simulink model "adm1"  (Simulink 6.1)
settings: Solver=ode15s  SolverMode=SingleTasking  StartTime=0.0  StopTime=600  MaxStep=0.5  RelTol=1e-6  AbsTol=1e-6
PreLoadFcn:
  | ADM1init
libraries: simulink x1
settings Model: Creator=ielulf  LastModifiedBy=evren.tugtas  ExtModeTrigMode=oneshot  ExtModeArmWhenConnect=off  ExtModeAutoUpdateStatusClock=off
settings DataIOCC: LimitDataPoints=off  SignalLoggingName=sigsOut
settings OptimizationCC: BlockReduction=off  BooleanDataType=off
settings HardwareCC: TargetUnknown=on
settings GRTTargetCC: ModelReferenceCompliant=off  MatFileLogging=off

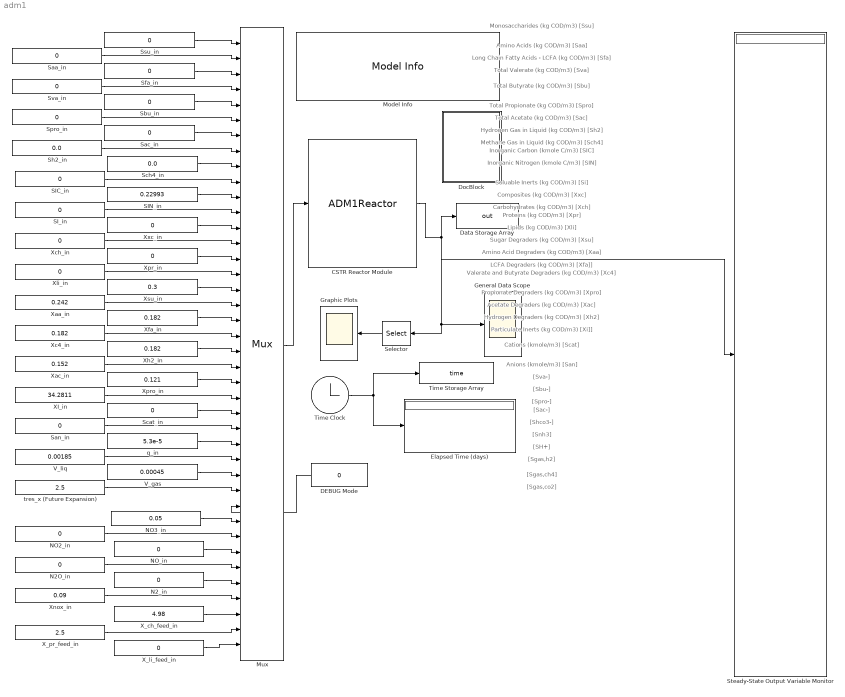
== system adm1 ==
  note: Monosaccharides (kg COD/m3) [Ssu]
  note: Amino Acids (kg COD/m3) [Saa]
  note: Long Chain Fatty Acids - LCFA (kg COD/m3) [Sfa]
  note: Total Valerate (kg COD/m3) [Sva]
  note: Total Butyrate (kg COD/m3) [Sbu]
  note: Total Propionate (kg COD/m3) [Spro]
  note: Total Acetate (kg COD/m3) [Sac]
  note: Hydrogen Gas in Liquid (kg COD/m3) [Sh2]
  note: Methane Gas in Liquid (kg COD/m3) [Sch4]
  note: Inorganic Carbon (kmole C/m3) [SIC]
  note: Inorganic Nitrogen (kmole C/m3) [SIN]
  note: Soluable Inerts (kg COD/m3) [Si]
  note: Composites (kg COD/m3) [Xxc]
  note: Carbohydrates (kg COD/m3) [Xch]
  note: Proteins (kg COD/m3) [Xpr]
  note: Lipids (kg COD/m3) [Xli]
  note: Amino Acid Degraders (kg COD/m3) [Xaa]
  note: LCFA Degraders (kg COD/m3) [Xfa]]
  note: Valerate and Butyrate Degraders (kg COD/m3) [Xc4]
  note: Propionate Degraders (kg COD/m3) [Xpro]
  note: Acetate Degraders (kg COD/m3) [Xac]
  note: Hydrogen Degraders (kg COD/m3) [Xh2]
  note: Particulate Inerts (kg COD/m3) [Xi]]
  note: Cations (kmole/m3) [Scat]
  note: Anions (kmole/m3) [San]
  note: [Sva-]
  note: [Sbu-]
  note: [Spro-]
  note: [Sac-]
  note: [Shco3-]
  note: [Snh3]
  note: [SH+]
  note: [Sgas,h2]
  note: [Sgas,ch4]
  note: [Sgas,co2]
  note: Sugar Degraders (kg COD/m3) [Xsu]
  CSTR Reactor Module : S-Function  FunctionName=ADM1Reactor
  DEBUG Mode : Constant  Tag=DEBUG  Orientation=left  Priority=0  Value=0  OutDataTypeMode=double
  Data Storage Array : ToWorkspace  VariableName=out  SampleTime=-1  SaveFormat=Array
      settings: Priority=14
  DocBlock : Subsystem  mask(DocBlock){ECoderFlag=, DocumentType=Text}
      mask prompts: ECoderFlag "E Coder Flag"; DocumentType "Document Type"
      mask help: Use this block to save long descriptive text with the model. Double-clicking the block will open an editor.
      settings: CopyFcn=docblock('breaklink',gcb);  DeleteFcn=docblock('close_document',gcb);  PreSaveFcn=docblock('save_document',gcb);  OpenFcn=docblock('edit_document',gcb);
      mask StyleString: edit,popup(Text|RTF|HTML)
      mask Display:
      | plot([.8 0 0 1 1 .8 .8 1],[1 1 0 0 .8 1 .8 .8]);
      | text(.5,.5,'DOC','horizontalalignment','center');
  Elapsed Time (days) : Display
      settings: Priority=4
  General Data Scope : Scope
      settings: TickLabels=on  YMin=0  YMax=50  SaveName=N1  DataFormat=Structure
  Graphic Plots : Scope
      settings: TickLabels=on  YMin=0.1  YMax=0.32  SaveName=N  DataFormat=Array
  Model Info : simulink/Model-Wide Utilities/Model Info  InitialBlockCM=none  BlockCM=none  Frame=on  DisplayStringWithTags=|  HorizontalTextAlignment=Left  LeftAlignmentValue=0.02  SourceBlockDiagram=adm1  TagMaxNumber=20
      | ADM1 Anaerobic Digestion Model %<Description>
      | Date Created: %<Created>
      | Date Last Modification: %<ModifiedDate>
      | Last Modified By: %<ModifiedBy>
      | ADM1 Model Version: %<ModelVersion>
      | ON-LINE DOCUMENTATION MANUAL  ===V=V=V=== %<ModifiedComment>
  Mux : Mux  Inputs=40
  N2O_in : Constant  Tag=N2O_in  Priority=0  Value=0  OutDataTypeMode=double
  N2_in : Constant  Tag=N2_in  Priority=0  Value=0  OutDataTypeMode=double
  NO2_in : Constant  Tag=NO2_in  Priority=0  Value=0  OutDataTypeMode=double
  NO3_in : Constant  Tag=NO3_in  Priority=0  Value=0.05  OutDataTypeMode=double
  NO_in : Constant  Tag=NO_in  Priority=0  Value=0  OutDataTypeMode=double
  SIC_in : Constant  Tag=SIC_in  Priority=0  Value=0  OutDataTypeMode=double
  SIN_in : Constant  Tag=SIN_in  Priority=0  Value=0.22993  OutDataTypeMode=double
  SI_in : Constant  Tag=SI_in  Priority=0  Value=0  OutDataTypeMode=double
  Saa_in : Constant  Tag=Saa_in  Priority=0  Value=0  OutDataTypeMode=double
  Sac_in : Constant  Tag=Sac_in  Priority=0  Value=0  OutDataTypeMode=double
  San_in : Constant  Tag=San_in  Priority=0  Value=0  OutDataTypeMode=double
  Sbu_in : Constant  Tag=Sbu_in  Priority=0  Value=0  OutDataTypeMode=double
  Scat_in : Constant  Priority=0  Value=0  OutDataTypeMode=double
  Sch4_in : Constant  Tag=Sch4_in  Priority=0  Value=0.0  OutDataTypeMode=double
  Selector : Selector  Orientation=left  Elements="[1  2  3  4  5  6  7]"  InputPortWidth=48
      settings: OpenFcn=ADM1Output
  Sfa_in : Constant  Tag=Sfa_in  Priority=0  Value=0  OutDataTypeMode=double
  Sh2_in : Constant  Tag=Sh2_in  Priority=0  Value=0.0  OutDataTypeMode=double
  Spro_in : Constant  Tag=Spro_in  Priority=0  Value=0  OutDataTypeMode=double
  Ssu_in : Constant  Tag=Ssu_in  Priority=0  Value=0  OutDataTypeMode=double
  Steady-State Output Variable Monitor : Display
      settings: Priority=2
  Sva_in : Constant  Tag=Sva_in  Priority=0  Value=0  OutDataTypeMode=double
  Time Clock : Clock
      settings: Priority=3  Decimation=10
  Time Storage Array : ToWorkspace  VariableName=time  SampleTime=-1  SaveFormat=Array
      settings: Priority=5
  V_gas : Constant  Tag=V_gas  Priority=0  Value=0.00045  OutDataTypeMode=double
  V_liq : Constant  Tag=V_liq  Priority=0  Value=0.00185  OutDataTypeMode=double
  XI_in : Constant  Tag=XI_in  Priority=0  Value=34.2811  OutDataTypeMode=double
  X_ch_feed_in : Constant  Tag=X_ch_feed_in  Priority=0  Value=4.98  OutDataTypeMode=double
  X_li_feed_in : Constant  Tag=X_li_feed_in  Priority=0  Value=0  OutDataTypeMode=double
  X_pr_feed_in : Constant  Tag=X_pr_feed_in  Priority=0  Value=2.5  OutDataTypeMode=double
  Xaa_in : Constant  Tag=Xaa_in  Priority=0  Value=0.242  OutDataTypeMode=double
  Xac_in : Constant  Tag=Xac_in  Priority=0  Value=0.152  OutDataTypeMode=double
  Xc4_in : Constant  Tag=Xc4_in  Priority=0  Value=0.182  OutDataTypeMode=double
  Xch_in : Constant  Tag=Xch_in  Priority=0  Value=0  OutDataTypeMode=double
  Xfa_in : Constant  Tag=Xfa_in  Priority=0  Value=0.182  OutDataTypeMode=double
  Xh2_in : Constant  Tag=Xh2_in  Priority=0  Value=0.182  OutDataTypeMode=double
  Xli_in : Constant  Tag=Xli_in  Priority=0  Value=0  OutDataTypeMode=double
  Xnox_in : Constant  Tag=Xnox_in  Priority=0  Value=0.09  OutDataTypeMode=double
  Xpr_in : Constant  Tag=Xpr_in  Priority=0  Value=0  OutDataTypeMode=double
  Xpro_in : Constant  Tag=Xpro_in  Priority=0  Value=0.121  OutDataTypeMode=double
  Xsu_in : Constant  Tag=Xsu_in  Priority=0  Value=0.3  OutDataTypeMode=double
  Xxc_in : Constant  Tag=Xxc_in  Priority=0  Value=0  OutDataTypeMode=double
  q_in : Constant  Tag=q_in  Priority=0  Value=5.3e-5  OutDataTypeMode=double
  "tres_x (Future Expansion) " : Constant  Tag=tres_x  Priority=0  Value=2.5  OutDataTypeMode=double
  wires:
  CSTR Reactor Module/1 -> Data Storage Array/1, Steady-State Output Variable Monitor/1, General Data Scope/1, Selector/1
  Time Clock/1 -> Time Storage Array/1, Elapsed Time (days)/1
  Ssu_in/1 -> Mux/1
  Saa_in/1 -> Mux/2
  Sfa_in/1 -> Mux/3
  Sva_in/1 -> Mux/4
  Sbu_in/1 -> Mux/5
  Spro_in/1 -> Mux/6
  Sac_in/1 -> Mux/7
  Sh2_in/1 -> Mux/8
  Sch4_in/1 -> Mux/9
  SIC_in/1 -> Mux/10
  SIN_in/1 -> Mux/11
  SI_in/1 -> Mux/12
  Xxc_in/1 -> Mux/13
  Xch_in/1 -> Mux/14
  Xpr_in/1 -> Mux/15
  Xli_in/1 -> Mux/16
  Xsu_in/1 -> Mux/17
  Xaa_in/1 -> Mux/18
  Xfa_in/1 -> Mux/19
  Xc4_in/1 -> Mux/20
  Xac_in/1 -> Mux/22
  XI_in/1 -> Mux/24
  Scat_in/1 -> Mux/25
  San_in/1 -> Mux/26
  q_in/1 -> Mux/27
  Mux/1 -> CSTR Reactor Module/1
  Xh2_in/1 -> Mux/21
  Xpro_in/1 -> Mux/23
  V_liq/1 -> Mux/28
  V_gas/1 -> Mux/29
  "tres_x (Future Expansion) "/1 -> Mux/30
  DEBUG Mode/1 -> Mux/31
  Selector/1 -> Graphic Plots/1
  NO3_in/1 -> Mux/32
  NO2_in/1 -> Mux/33
  NO_in/1 -> Mux/34
  N2O_in/1 -> Mux/35
  N2_in/1 -> Mux/36
  Xnox_in/1 -> Mux/37
  X_ch_feed_in/1 -> Mux/38
  X_pr_feed_in/1 -> Mux/39
  X_li_feed_in/1 -> Mux/40

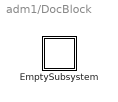
== system adm1/DocBlock ==
  EmptySubsystem : Subsystem

== system adm1/DocBlock/EmptySubsystem ==
